simulink model "conbloques"  (Simulink 7.6)
settings: Solver=ode45  StartTime=0.0  StopTime=20.0  RelTol=0.01
settings Model: Creator=spaterna  LastModifiedBy=pater  ExtModeAutoUpdateStatusClock=off
settings SolverCC: MaxConsecutiveMinStep=10
settings OptimizationCC: InitFltsAndDblsToZero=on
settings DebuggingCC: SaveWithParameterizedLinksMsg=none  StrictBusMsg=Warning
settings GRTTargetCC: TargetFcnLib=ansi_tfl_tmw.mat

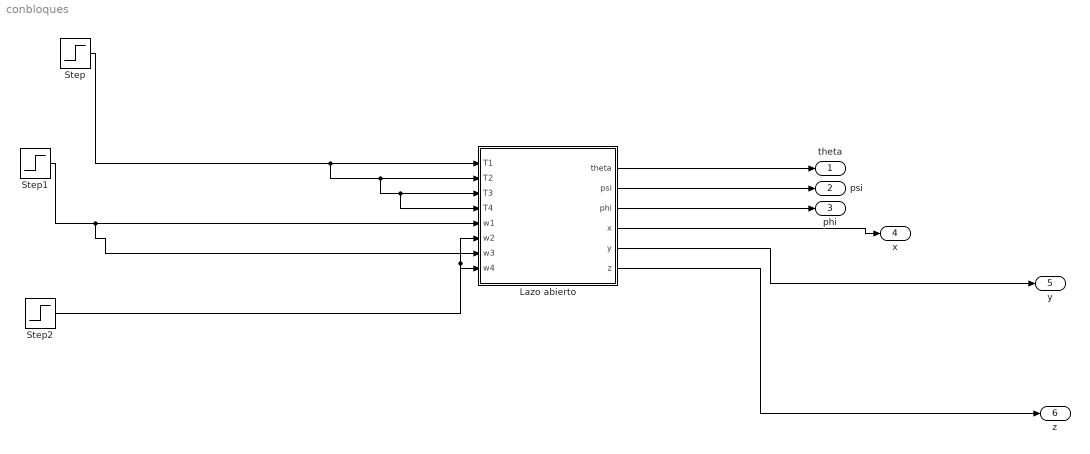
== system conbloques ==
  Lazo abierto : Subsystem
  Step : Step  Before=2.45  After=2.45  SampleTime=0
  Step1 : Step  Before=5  After=5  SampleTime=0
  Step2 : Step  Time=5  Before=-5  After=-2.5  SampleTime=0
  theta : Outport
  psi : Outport  Port=2
  phi : Outport  Port=3
  x : Outport  Port=4
  y : Outport  Port=5
  z : Outport  Port=6
  wires:
  Lazo abierto/1(theta) -> theta/1
  Lazo abierto/2(psi) -> psi/1
  Step/1 -> Lazo abierto/1(T1), Lazo abierto/2(T2), Lazo abierto/3(T3), Lazo abierto/4(T4)
  Lazo abierto/4(x) -> x/1
  Lazo abierto/5(y) -> y/1
  Lazo abierto/6(z) -> z/1
  Step1/1 -> Lazo abierto/5(w1), Lazo abierto/7(w3)
  Lazo abierto/3(phi) -> phi/1
  Step2/1 -> Lazo abierto/6(w2), Lazo abierto/8(w4)

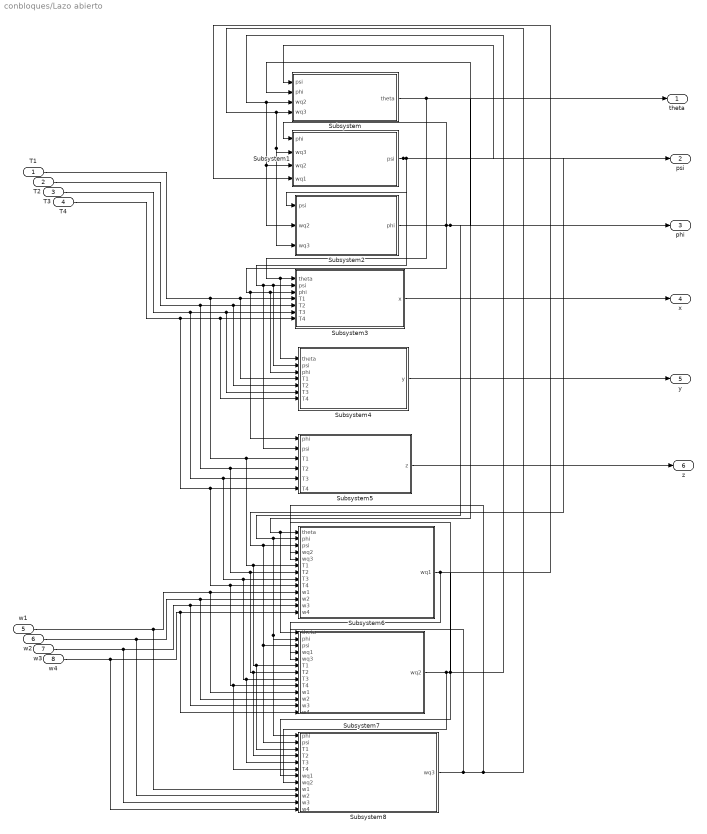
== system conbloques/Lazo abierto ==
  T1 : Inport
  T2 : Inport  Port=2
  T3 : Inport  Port=3
  T4 : Inport  Port=4
  w1 : Inport  Port=5
  w2 : Inport  Port=6
  w3 : Inport  Port=7
  w4 : Inport  Port=8
  Subsystem : Subsystem
  Subsystem1 : Subsystem
  Subsystem2 : Subsystem
  Subsystem3 : Subsystem
  Subsystem4 : Subsystem
  Subsystem5 : Subsystem
  Subsystem6 : Subsystem
  Subsystem7 : Subsystem
  Subsystem8 : Subsystem
  theta : Outport
  psi : Outport  Port=2
  phi : Outport  Port=3
  x : Outport  Port=4
  y : Outport  Port=5
  z : Outport  Port=6
  wires:
  Subsystem7/1(wq2) -> Subsystem6/4(wq2), Subsystem/3(wq2), Subsystem1/3(wq2), Subsystem2/2(wq2), Subsystem8/8(wq2)
  Subsystem8/1(wq3) -> Subsystem6/5(wq3), Subsystem/4(wq3), Subsystem1/2(wq3), Subsystem2/3(wq3), Subsystem7/5(wq3)
  Subsystem6/1(wq1) -> Subsystem7/4(wq1), Subsystem8/7(wq1), Subsystem1/4(wq1)
  w1/1 -> Subsystem6/10(w1), Subsystem7/10(w1), Subsystem8/9(w1)
  w2/1 -> Subsystem6/11(w2), Subsystem7/11(w2), Subsystem8/10(w2)
  w3/1 -> Subsystem6/12(w3), Subsystem7/12(w3), Subsystem8/11(w3)
  w4/1 -> Subsystem6/13(w4), Subsystem7/13(w4), Subsystem8/12(w4)
  Subsystem5/1(z) -> z/1
  Subsystem4/1(y) -> y/1
  Subsystem3/1(x) -> x/1
  Subsystem/1(theta) -> Subsystem3/1(theta), Subsystem4/1(theta), theta/1, Subsystem6/1(theta), Subsystem7/1(theta)
  T4/1 -> Subsystem3/7(T4), Subsystem4/7(T4), Subsystem5/6(T4), Subsystem6/9(T4), Subsystem7/9(T4), Subsystem8/6(T4)
  T3/1 -> Subsystem3/6(T3), Subsystem4/6(T3), Subsystem5/5(T3), Subsystem6/8(T3), Subsystem7/8(T3), Subsystem8/5(T3)
  T2/1 -> Subsystem3/5(T2), Subsystem4/5(T2), Subsystem5/4(T2), Subsystem6/7(T2), Subsystem7/7(T2), Subsystem8/4(T2)
  T1/1 -> Subsystem3/4(T1), Subsystem4/4(T1), Subsystem5/3(T1), Subsystem6/6(T1), Subsystem7/6(T1), Subsystem8/3(T1)
  Subsystem2/1(phi) -> Subsystem1/1(phi), Subsystem3/3(phi), Subsystem4/3(phi), Subsystem5/1(phi), Subsystem/2(phi), phi/1, Subsystem6/2(phi), Subsystem7/2(phi), Subsystem8/1(phi)
  Subsystem1/1(psi) -> Subsystem/1(psi), Subsystem2/1(psi), Subsystem3/2(psi), Subsystem4/2(psi), Subsystem5/2(psi), psi/1, Subsystem6/3(psi), Subsystem7/3(psi), Subsystem8/2(psi)

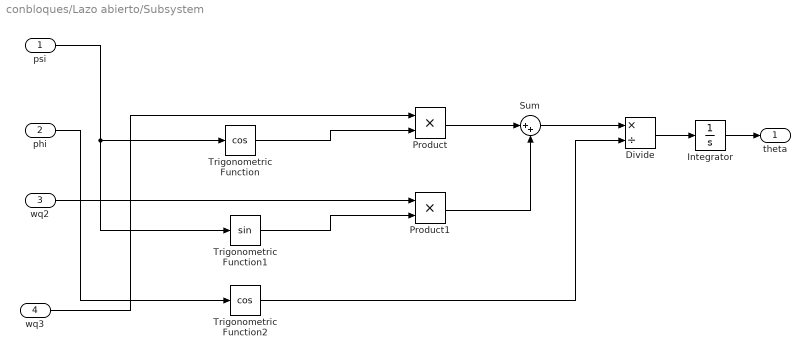
== system conbloques/Lazo abierto/Subsystem ==
  psi : Inport
  phi : Inport  Port=2
  wq2 : Inport  Port=3
  wq3 : Inport  Port=4
  Divide : Product  Inputs=*/
  Integrator : Integrator
  Product : Product  RndMeth=Zero
  Product1 : Product  RndMeth=Zero
  Sum : Sum  Inputs=|++
  Trigonometric Function : Trigonometry  Operator=cos
  Trigonometric Function1 : Trigonometry
  Trigonometric Function2 : Trigonometry  Operator=cos
  theta : Outport
  wires:
  wq3/1 -> Product/1
  wq2/1 -> Product1/1
  Product/1 -> Sum/1
  Product1/1 -> Sum/2
  Sum/1 -> Divide/1
  Trigonometric Function2/1 -> Divide/2
  Divide/1 -> Integrator/1
  Trigonometric Function/1 -> Product/2
  Trigonometric Function1/1 -> Product1/2
  phi/1 -> Trigonometric Function2/1
  Integrator/1 -> theta/1
  psi/1 -> Trigonometric Function/1, Trigonometric Function1/1

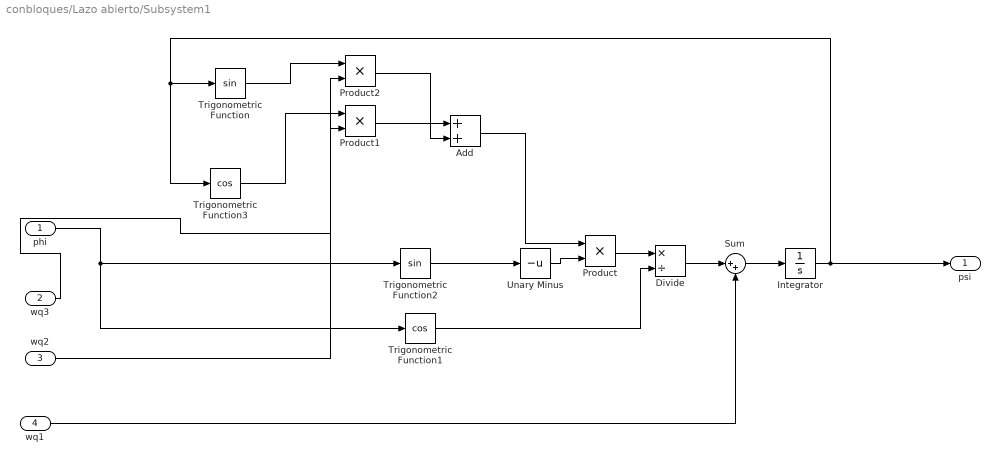
== system conbloques/Lazo abierto/Subsystem1 ==
  phi : Inport
  wq3 : Inport  Port=2
  wq2 : Inport  Port=3
  wq1 : Inport  Port=4
  Add : Sum
  Divide : Product  Inputs=*/
  Integrator : Integrator
  Product : Product  RndMeth=Zero
  Product1 : Product  RndMeth=Zero
  Product2 : Product  RndMeth=Zero
  Sum : Sum  Inputs=|++
  Trigonometric Function : Trigonometry
  Trigonometric Function1 : Trigonometry  Operator=cos
  Trigonometric Function2 : Trigonometry
  Trigonometric Function3 : Trigonometry  Operator=cos
  Unary Minus : UnaryMinus
  psi : Outport
  wires:
  Integrator/1 -> psi/1, Trigonometric Function3/1, Trigonometric Function/1
  Product/1 -> Divide/1
  Trigonometric Function1/1 -> Divide/2
  phi/1 -> Trigonometric Function1/1, Trigonometric Function2/1
  Trigonometric Function2/1 -> Unary Minus/1
  Unary Minus/1 -> Product/2
  wq3/1 -> Product1/2
  Trigonometric Function3/1 -> Product1/1
  Product1/1 -> Add/1
  Add/1 -> Product/1
  Trigonometric Function/1 -> Product2/1
  wq2/1 -> Product2/2
  Product2/1 -> Add/2
  Divide/1 -> Sum/1
  wq1/1 -> Sum/2
  Sum/1 -> Integrator/1

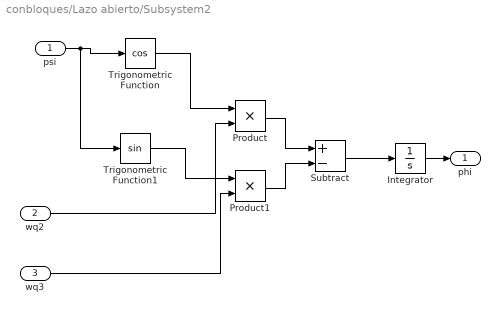
== system conbloques/Lazo abierto/Subsystem2 ==
  psi : Inport
  wq2 : Inport  Port=2
  wq3 : Inport  Port=3
  Integrator : Integrator
  Product : Product  RndMeth=Zero
  Product1 : Product  RndMeth=Zero
  Subtract : Sum  Inputs=+-
  Trigonometric Function : Trigonometry  Operator=cos
  Trigonometric Function1 : Trigonometry
  phi : Outport
  wires:
  Integrator/1 -> phi/1
  Subtract/1 -> Integrator/1
  Product/1 -> Subtract/1
  Product1/1 -> Subtract/2
  Trigonometric Function/1 -> Product/1
  psi/1 -> Trigonometric Function/1, Trigonometric Function1/1
  Trigonometric Function1/1 -> Product1/1
  wq2/1 -> Product/2
  wq3/1 -> Product1/2

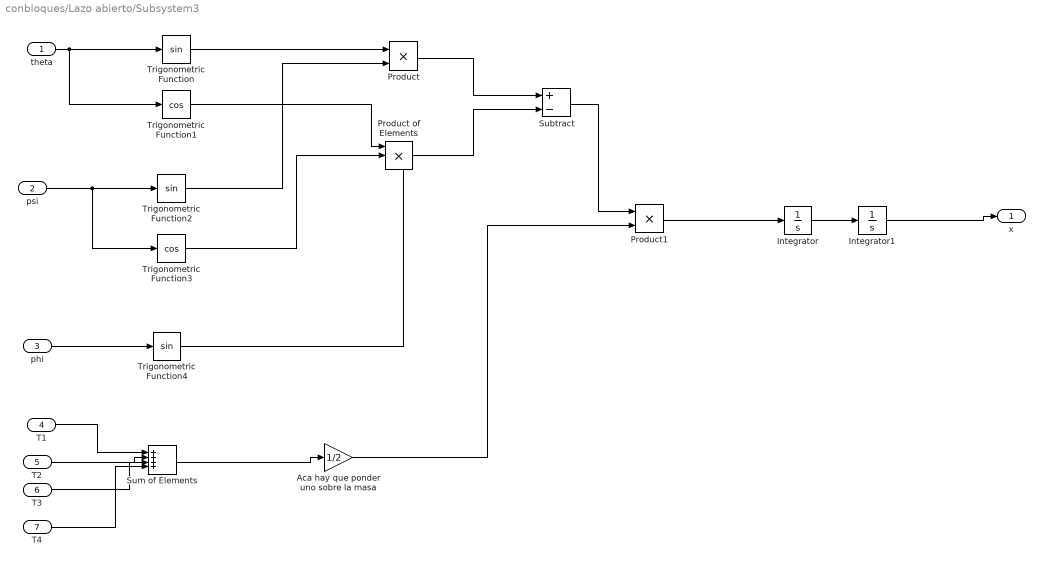
== system conbloques/Lazo abierto/Subsystem3 ==
  theta : Inport
  psi : Inport  Port=2
  phi : Inport  Port=3
  T1 : Inport  Port=4
  T2 : Inport  Port=5
  T3 : Inport  Port=6
  T4 : Inport  Port=7
  Aca hay que ponder uno sobre la masa : Gain  Gain=1/2
  Integrator : Integrator
  Integrator1 : Integrator
  Product : Product  RndMeth=Zero
  Product of Elements : Product  Inputs=3
  Product1 : Product  RndMeth=Zero
  Subtract : Sum  Inputs=+-
  Sum of Elements : Sum  Inputs=4
  Trigonometric Function : Trigonometry
  Trigonometric Function1 : Trigonometry  Operator=cos
  Trigonometric Function2 : Trigonometry
  Trigonometric Function3 : Trigonometry  Operator=cos
  Trigonometric Function4 : Trigonometry
  x : Outport
  wires:
  theta/1 -> Trigonometric Function/1, Trigonometric Function1/1
  psi/1 -> Trigonometric Function2/1, Trigonometric Function3/1
  phi/1 -> Trigonometric Function4/1
  Trigonometric Function/1 -> Product/1
  Trigonometric Function2/1 -> Product/2
  Trigonometric Function1/1 -> Product of Elements/1
  Trigonometric Function3/1 -> Product of Elements/2
  Trigonometric Function4/1 -> Product of Elements/3
  Product/1 -> Subtract/1
  Product of Elements/1 -> Subtract/2
  Product1/1 -> Integrator/1
  T1/1 -> Sum of Elements/1
  T2/1 -> Sum of Elements/2
  T4/1 -> Sum of Elements/4
  T3/1 -> Sum of Elements/3
  Sum of Elements/1 -> Aca hay que ponder uno sobre la masa/1
  Aca hay que ponder uno sobre la masa/1 -> Product1/2
  Subtract/1 -> Product1/1
  Integrator/1 -> Integrator1/1
  Integrator1/1 -> x/1

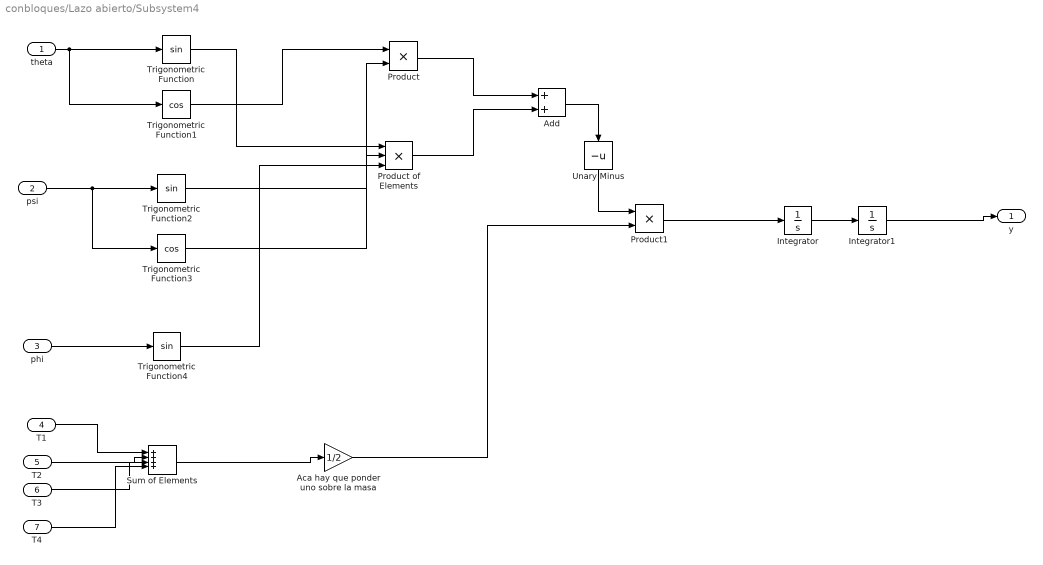
== system conbloques/Lazo abierto/Subsystem4 ==
  theta : Inport
  psi : Inport  Port=2
  phi : Inport  Port=3
  T1 : Inport  Port=4
  T2 : Inport  Port=5
  T3 : Inport  Port=6
  T4 : Inport  Port=7
  Aca hay que ponder uno sobre la masa : Gain  Gain=1/2
  Add : Sum
  Integrator : Integrator
  Integrator1 : Integrator
  Product : Product  RndMeth=Zero
  Product of Elements : Product  Inputs=3
  Product1 : Product  RndMeth=Zero
  Sum of Elements : Sum  Inputs=4
  Trigonometric Function : Trigonometry
  Trigonometric Function1 : Trigonometry  Operator=cos
  Trigonometric Function2 : Trigonometry
  Trigonometric Function3 : Trigonometry  Operator=cos
  Trigonometric Function4 : Trigonometry
  Unary Minus : UnaryMinus
  y : Outport
  wires:
  theta/1 -> Trigonometric Function/1, Trigonometric Function1/1
  psi/1 -> Trigonometric Function2/1, Trigonometric Function3/1
  phi/1 -> Trigonometric Function4/1
  Product/1 -> Add/1
  Product of Elements/1 -> Add/2
  Product1/1 -> Integrator/1
  T1/1 -> Sum of Elements/1
  T2/1 -> Sum of Elements/2
  T4/1 -> Sum of Elements/4
  T3/1 -> Sum of Elements/3
  Sum of Elements/1 -> Aca hay que ponder uno sobre la masa/1
  Aca hay que ponder uno sobre la masa/1 -> Product1/2
  Add/1 -> Unary Minus/1
  Integrator/1 -> Integrator1/1
  Integrator1/1 -> y/1
  Trigonometric Function2/1 -> Product/2
  Trigonometric Function1/1 -> Product/1
  Trigonometric Function/1 -> Product of Elements/1
  Trigonometric Function3/1 -> Product of Elements/2
  Trigonometric Function4/1 -> Product of Elements/3
  Unary Minus/1 -> Product1/1

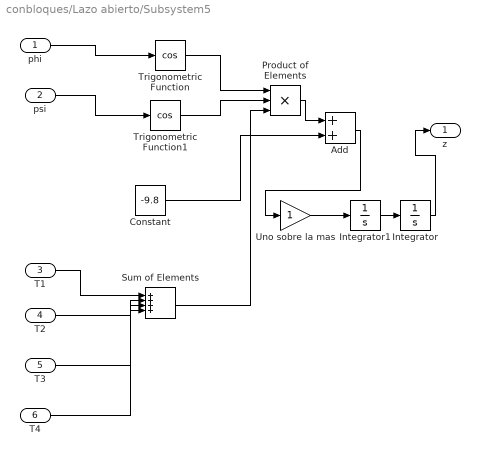
== system conbloques/Lazo abierto/Subsystem5 ==
  phi : Inport
  psi : Inport  Port=2
  T1 : Inport  Port=3
  T2 : Inport  Port=4
  T3 : Inport  Port=5
  T4 : Inport  Port=6
  Add : Sum
  Constant : Constant  Value=-9.8
  Integrator : Integrator
  Integrator1 : Integrator
  Product of Elements : Product  Inputs=3
  Sum of Elements : Sum  Inputs=4
  Trigonometric Function : Trigonometry  Operator=cos
  Trigonometric Function1 : Trigonometry  Operator=cos
  Uno sobre la mas : Gain
  z : Outport
  wires:
  T1/1 -> Sum of Elements/1
  T2/1 -> Sum of Elements/2
  T3/1 -> Sum of Elements/3
  T4/1 -> Sum of Elements/4
  phi/1 -> Trigonometric Function/1
  psi/1 -> Trigonometric Function1/1
  Trigonometric Function/1 -> Product of Elements/1
  Trigonometric Function1/1 -> Product of Elements/2
  Sum of Elements/1 -> Product of Elements/3
  Uno sobre la mas/1 -> Integrator1/1
  Integrator1/1 -> Integrator/1
  Integrator/1 -> z/1
  Product of Elements/1 -> Add/1
  Constant/1 -> Add/2
  Add/1 -> Uno sobre la mas/1

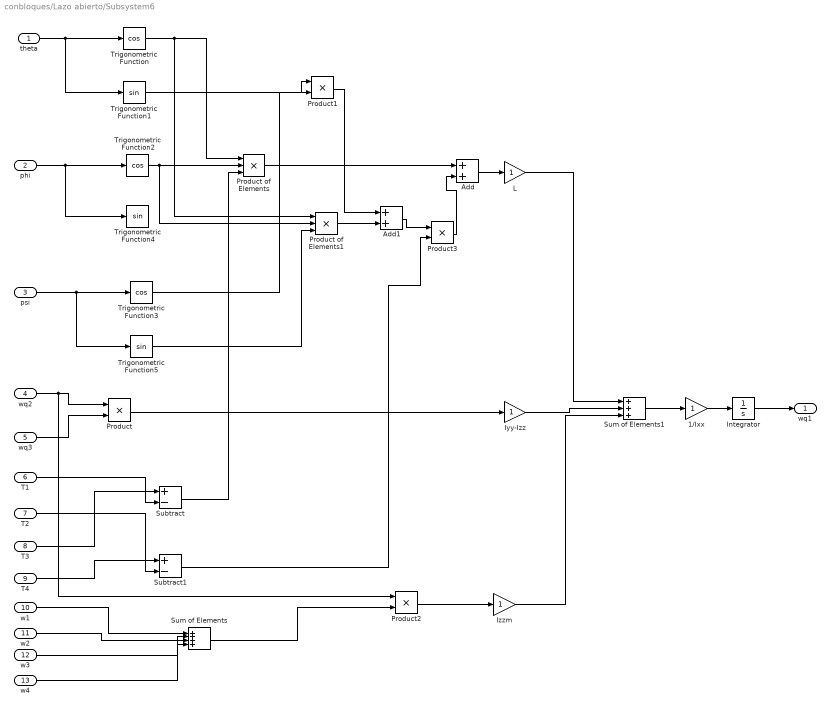
== system conbloques/Lazo abierto/Subsystem6 ==
  theta : Inport
  phi : Inport  Port=2
  psi : Inport  Port=3
  wq2 : Inport  Port=4
  wq3 : Inport  Port=5
  T1 : Inport  Port=6
  T2 : Inport  Port=7
  T3 : Inport  Port=8
  T4 : Inport  Port=9
  w1 : Inport  Port=10
  w2 : Inport  Port=11
  w3 : Inport  Port=12
  w4 : Inport  Port=13
  1/Ixx : Gain
  Add : Sum
  Add1 : Sum
  Integrator : Integrator
  Iyy-Izz : Gain
  Izzm : Gain
  L : Gain
  Product{,1..3} (4 alike) : Product  RndMeth=Zero
  Product of Elements : Product  Inputs=3
  Product of Elements1 : Product  Inputs=3
  Subtract : Sum  Inputs=+-
  Subtract1 : Sum  Inputs=+-
  Sum of Elements : Sum  Inputs=4
  Sum of Elements1 : Sum  Inputs=3
  Trigonometric Function : Trigonometry  Operator=cos
  Trigonometric Function1 : Trigonometry
  Trigonometric Function2 : Trigonometry  Operator=cos
  Trigonometric Function3 : Trigonometry  Operator=cos
  Trigonometric Function4 : Trigonometry
  Trigonometric Function5 : Trigonometry
  wq1 : Outport
  wires:
  theta/1 -> Trigonometric Function/1, Trigonometric Function1/1
  phi/1 -> Trigonometric Function2/1, Trigonometric Function4/1
  psi/1 -> Trigonometric Function3/1, Trigonometric Function5/1
  wq2/1 -> Product/1, Product2/1
  wq3/1 -> Product/2
  Product/1 -> Iyy-Izz/1
  Trigonometric Function/1 -> Product of Elements/1, Product of Elements1/1
  Trigonometric Function2/1 -> Product of Elements/2, Product of Elements1/2
  T3/1 -> Subtract/1
  T1/1 -> Subtract/2
  Subtract/1 -> Product of Elements/3
  Trigonometric Function1/1 -> Product1/1
  Trigonometric Function3/1 -> Product1/2
  Trigonometric Function5/1 -> Product of Elements1/3
  T4/1 -> Subtract1/1
  T2/1 -> Subtract1/2
  Subtract1/1 -> Product3/2
  Product1/1 -> Add1/1
  Product of Elements/1 -> Add/1
  Add/1 -> L/1
  w1/1 -> Sum of Elements/1
  w2/1 -> Sum of Elements/2
  w3/1 -> Sum of Elements/3
  w4/1 -> Sum of Elements/4
  Sum of Elements/1 -> Product2/2
  Product2/1 -> Izzm/1
  L/1 -> Sum of Elements1/1
  Iyy-Izz/1 -> Sum of Elements1/2
  Izzm/1 -> Sum of Elements1/3
  Sum of Elements1/1 -> 1/Ixx/1
  1/Ixx/1 -> Integrator/1
  Integrator/1 -> wq1/1
  Product of Elements1/1 -> Add1/2
  Add1/1 -> Product3/1
  Product3/1 -> Add/2

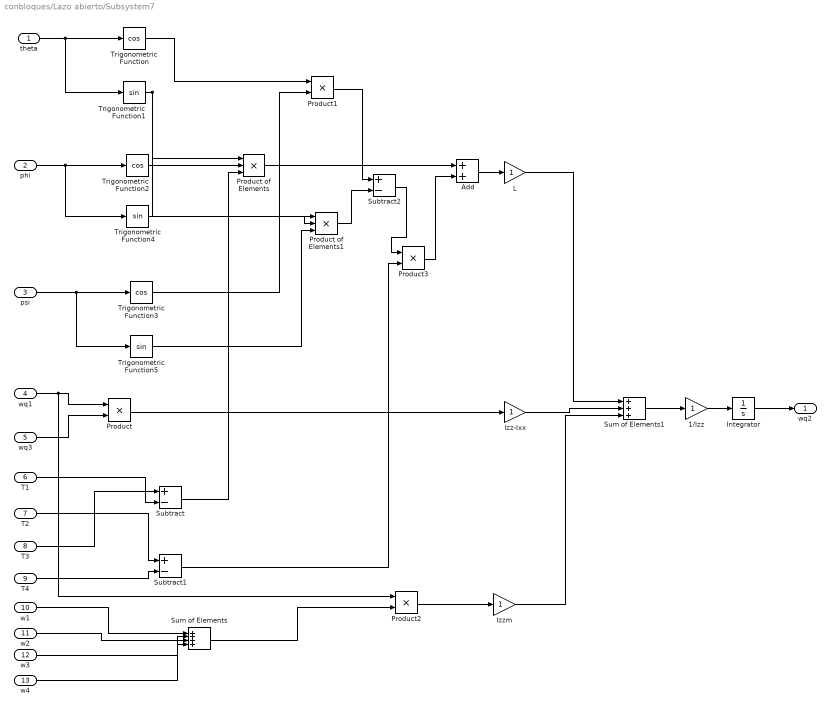
== system conbloques/Lazo abierto/Subsystem7 ==
  theta : Inport
  phi : Inport  Port=2
  psi : Inport  Port=3
  wq1 : Inport  Port=4
  wq3 : Inport  Port=5
  T1 : Inport  Port=6
  T2 : Inport  Port=7
  T3 : Inport  Port=8
  T4 : Inport  Port=9
  w1 : Inport  Port=10
  w2 : Inport  Port=11
  w3 : Inport  Port=12
  w4 : Inport  Port=13
  1/Izz : Gain
  Add : Sum
  Integrator : Integrator
  Izz-Ixx : Gain
  Izzm : Gain
  L : Gain
  Product{,1..3} (4 alike) : Product  RndMeth=Zero
  Product of Elements : Product  Inputs=3
  Product of Elements1 : Product  Inputs=3
  Subtract : Sum  Inputs=+-
  Subtract1 : Sum  Inputs=+-
  Subtract2 : Sum  Inputs=+-
  Sum of Elements : Sum  Inputs=4
  Sum of Elements1 : Sum  Inputs=3
  Trigonometric Function : Trigonometry  Operator=cos
  Trigonometric Function1 : Trigonometry
  Trigonometric Function2 : Trigonometry  Operator=cos
  Trigonometric Function3 : Trigonometry  Operator=cos
  Trigonometric Function4 : Trigonometry
  Trigonometric Function5 : Trigonometry
  wq2 : Outport
  wires:
  theta/1 -> Trigonometric Function/1, Trigonometric Function1/1
  phi/1 -> Trigonometric Function2/1, Trigonometric Function4/1
  psi/1 -> Trigonometric Function3/1, Trigonometric Function5/1
  wq1/1 -> Product/1, Product2/1
  wq3/1 -> Product/2
  Product/1 -> Izz-Ixx/1
  Trigonometric Function/1 -> Product1/1
  Trigonometric Function2/1 -> Product of Elements/2
  T3/1 -> Subtract/1
  T1/1 -> Subtract/2
  Subtract/1 -> Product of Elements/3
  Trigonometric Function1/1 -> Product of Elements/1, Product of Elements1/1
  Trigonometric Function3/1 -> Product1/2
  Trigonometric Function5/1 -> Product of Elements1/3
  Subtract1/1 -> Product3/2
  Product3/1 -> Add/2
  Product of Elements/1 -> Add/1
  Add/1 -> L/1
  w1/1 -> Sum of Elements/1
  w2/1 -> Sum of Elements/2
  w3/1 -> Sum of Elements/3
  w4/1 -> Sum of Elements/4
  Sum of Elements/1 -> Product2/2
  Product2/1 -> Izzm/1
  L/1 -> Sum of Elements1/1
  Izz-Ixx/1 -> Sum of Elements1/2
  Izzm/1 -> Sum of Elements1/3
  Sum of Elements1/1 -> 1/Izz/1
  1/Izz/1 -> Integrator/1
  Integrator/1 -> wq2/1
  Trigonometric Function4/1 -> Product of Elements1/2
  Product1/1 -> Subtract2/1
  Product of Elements1/1 -> Subtract2/2
  Subtract2/1 -> Product3/1
  T2/1 -> Subtract1/1
  T4/1 -> Subtract1/2

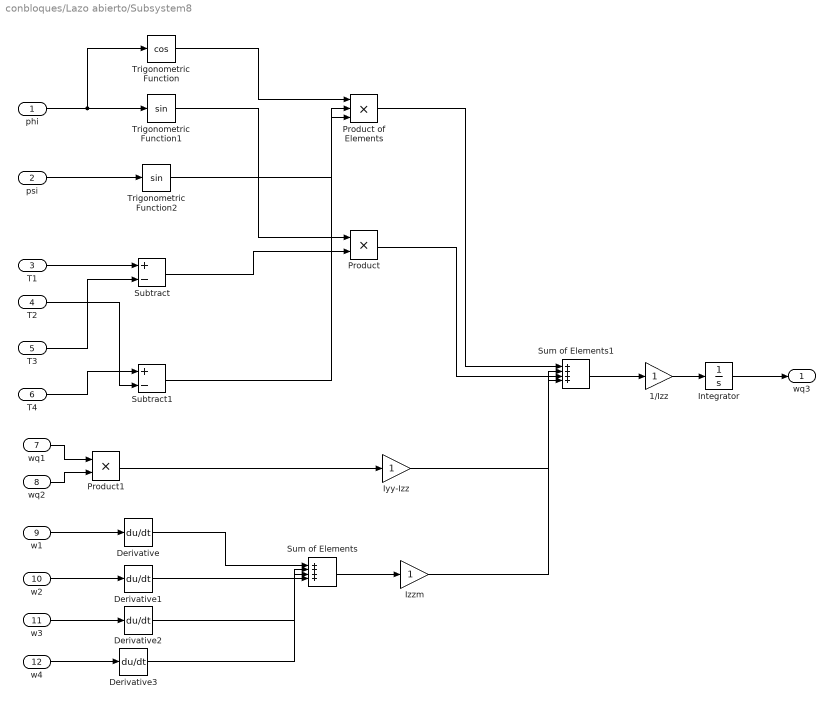
== system conbloques/Lazo abierto/Subsystem8 ==
  phi : Inport
  psi : Inport  Port=2
  T1 : Inport  Port=3
  T2 : Inport  Port=4
  T3 : Inport  Port=5
  T4 : Inport  Port=6
  wq1 : Inport  Port=7
  wq2 : Inport  Port=8
  w1 : Inport  Port=9
  w2 : Inport  Port=10
  w3 : Inport  Port=11
  w4 : Inport  Port=12
  1/Izz : Gain
  Derivative{,1..3} (4 alike) : Derivative
  Integrator : Integrator
  Iyy-Izz : Gain
  Izzm : Gain
  Product : Product  RndMeth=Zero
  Product of Elements : Product  Inputs=3
  Product1 : Product  RndMeth=Zero
  Subtract : Sum  Inputs=+-
  Subtract1 : Sum  Inputs=+-
  Sum of Elements : Sum  Inputs=4
  Sum of Elements1 : Sum  Inputs=4
  Trigonometric Function : Trigonometry  Operator=cos
  Trigonometric Function1 : Trigonometry
  Trigonometric Function2 : Trigonometry
  wq3 : Outport
  wires:
  phi/1 -> Trigonometric Function1/1, Trigonometric Function/1
  psi/1 -> Trigonometric Function2/1
  T1/1 -> Subtract/1
  T3/1 -> Subtract/2
  T4/1 -> Subtract1/1
  T2/1 -> Subtract1/2
  Trigonometric Function1/1 -> Product/1
  Subtract/1 -> Product/2
  Trigonometric Function/1 -> Product of Elements/1
  Trigonometric Function2/1 -> Product of Elements/2
  Subtract1/1 -> Product of Elements/3
  wq1/1 -> Product1/1
  wq2/1 -> Product1/2
  Product1/1 -> Iyy-Izz/1
  w4/1 -> Derivative3/1
  w3/1 -> Derivative2/1
  w2/1 -> Derivative1/1
  w1/1 -> Derivative/1
  Derivative/1 -> Sum of Elements/1
  Derivative1/1 -> Sum of Elements/2
  Derivative2/1 -> Sum of Elements/3
  Derivative3/1 -> Sum of Elements/4
  Sum of Elements/1 -> Izzm/1
  Product of Elements/1 -> Sum of Elements1/1
  Product/1 -> Sum of Elements1/2
  Iyy-Izz/1 -> Sum of Elements1/3
  Izzm/1 -> Sum of Elements1/4
  Sum of Elements1/1 -> 1/Izz/1
  1/Izz/1 -> Integrator/1
  Integrator/1 -> wq3/1
